simulink model "EmergencyBraking"  (R2023b)
settings: Solver=FixedStepAuto  StartTime=0.0  StopTime=inf  RelTol=1e-3
model workspace (MAT data in the model file):
  SL_ROS_VariableLengthArrays_MaxSizes.CommonInfo.ArrayTruncateAction = 'EmitWarning'
  SL_ROS_VariableLengthArrays_MaxSizes.MsgTypeMap = containers.Map
  SL_ROS_VariableLengthArrays_MaxSizes.MsgTypeMap.serialization.keys = {'sensor_msgs/PointCloud2'}
  SL_ROS_VariableLengthArrays_MaxSizes.MsgTypeMap.serialization.values{1}(1).PropertyName = 'data'
  SL_ROS_VariableLengthArrays_MaxSizes.MsgTypeMap.serialization.values{1}(1).DataType = 'uint8'
  SL_ROS_VariableLengthArrays_MaxSizes.MsgTypeMap.serialization.values{1}(1).MaxLength = 140000
  SL_ROS_VariableLengthArrays_MaxSizes.MsgTypeMap.serialization.values{1}(2).PropertyName = 'fields'
  SL_ROS_VariableLengthArrays_MaxSizes.MsgTypeMap.serialization.values{1}(2).DataType = 'sensor_msgs/PointField'
  SL_ROS_VariableLengthArrays_MaxSizes.MsgTypeMap.serialization.values{1}(2).MaxLength = 16
  SL_ROS_VariableLengthArrays_MaxSizes.MsgTypeMap.serialization.uniformity = 0
  SL_ROS_VariableLengthArrays_MaxSizes.MsgTypeMap.serialization.keyType = 'char'
  SL_ROS_VariableLengthArrays_MaxSizes.MsgTypeMap.serialization.valueType = 'any'
undefined symbols (not defined in the file): brake, throttle
libraries: ros2lib x5
settings Model: Creator=nikos  LastModifiedBy=nikos
settings OptimizationCC: EnhancedBackFolding=on  PassReuseOutputArgsAs=Individual arguments  ZeroExternalMemoryAtStartup=off  ZeroInternalMemoryAtStartup=off  MaxStackSize=64  OptimizeBlockOrder=speed  DifferentSizesBufferReuse=on  OptimizationCustomize=off  EfficientTunableParamExpr=on
settings DebuggingCC: ParameterTunabilityLossMsg=error
settings HardwareCC: ProdBitPerLong=64  ProdHWDeviceType=Intel->x86-64 (Linux 64)  UseEmbeddedCoderFeatures=off
settings SFSimCC: MATLABDynamicMemAlloc=off
settings RTWCC: Description=Embedded Coder  SystemTargetFile=ert.tlc  HardwareBoard=Robot Operating System 2 (ROS 2)  TLCOptions="-aInlineSetEventsForThisBaseRateFcn=TLC_FALSE -aSuppressMultiTaskScheduler=TLC_FALSE  -aRateBasedStepFcn=0"  TemplateMakefile=ert_default_tmf  Toolchain=Colcon Tools  TargetLang=C++
settings CodeAppCC: ForceParamTrailComments=on  IgnoreCustomStorageClasses=off  OperatorAnnotations=on  SimulinkDataObjDesc=on  SFDataObjDesc=on  InsertBlockDesc=on
settings ERTTargetCC: CodeInterfacePackaging=C++ class  SupportNonInlinedSFcns=on  RootIOFormat=Structure reference

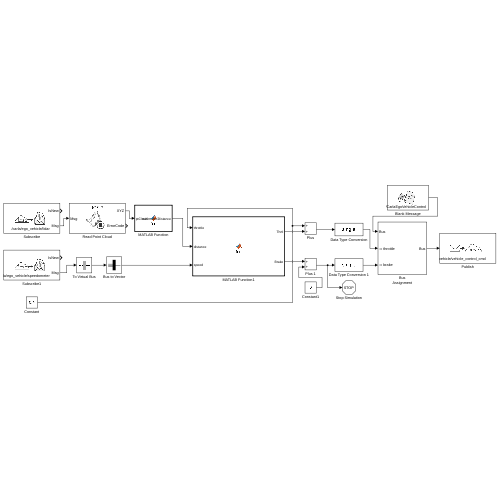
[thumbnail: Simulink's stored preview of the top-level diagram]
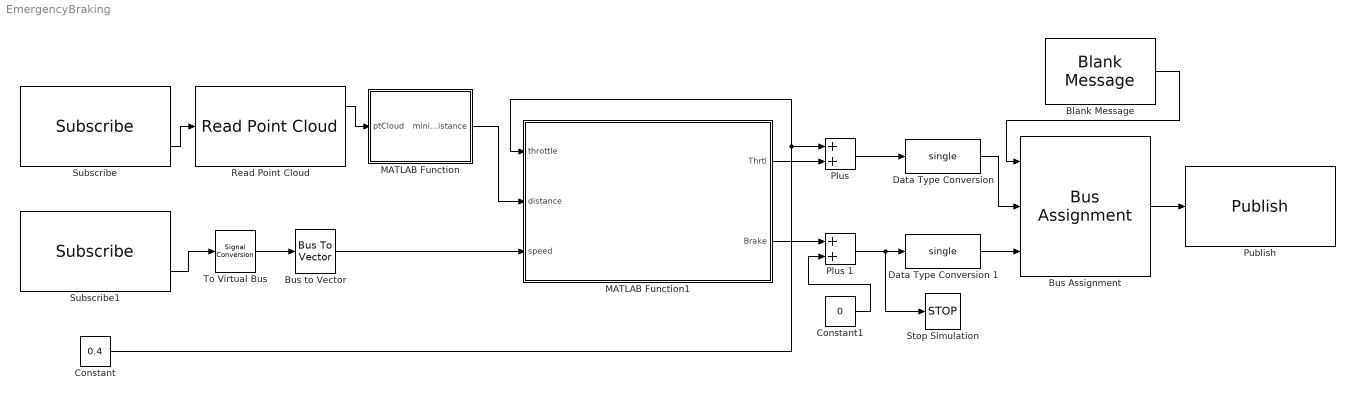
== system EmergencyBraking ==
  Blank Message : ros2lib/Blank Message  messageClass=Message  entityType=carla_msgs/CarlaEgoVehicleControl  messageType=carla_msgs/CarlaEgoVehicleControl  SampleTime=inf
  Bus Assignment : BusAssignment  AssignedSignals=throttle,brake
  Bus to Vector : BusToVector
  Constant : Constant  Value=0.4
  Constant1 : Constant  Value=0
  Data Type Conversion : DataTypeConversion  OutDataTypeStr=single  SaturateOnIntegerOverflow=off  RndMeth=Floor
  Data Type Conversion 1 : DataTypeConversion  OutDataTypeStr=single  SaturateOnIntegerOverflow=off  RndMeth=Floor
  MATLAB Function : MATLAB Function  TreatAsAtomicUnit=on
  MATLAB Function1 : MATLAB Function  TreatAsAtomicUnit=on
  Plus : Sum
  Plus 1 : Sum
  Publish : ros2lib/Publish  topicSource=Select from ROS network  topic=/carla/ego_vehicle/vehicle_control_cmd  messageType=carla_msgs/CarlaEgoVehicleControl  QOSHistory=Keep last  QOSDepth=1  QOSReliability=Reliable  QOSDurability=Volatile
  Read Point Cloud : ros2lib/Read Point Cloud  MaximumPointCloudSize=[480, 640]  PreserveStructure=off  ShowRGBOutput=off  ShowIntensityOutput=off  ShowErrorCodeOutput=on  VariableSizeOutputs=off
  Stop Simulation : Stop
  Subscribe : ros2lib/Subscribe  topicSource=Select from ROS network  topic=/carla/ego_vehicle/lidar  messageType=sensor_msgs/PointCloud2  sampleTime=-1  QOSHistory=Keep last  QOSDepth=1  QOSReliability=Reliable  QOSDurability=Volatile
  Subscribe1 : ros2lib/Subscribe  topicSource=Select from ROS network  topic=/carla/ego_vehicle/speedometer  messageType=std_msgs/Float32  sampleTime=-1  QOSHistory=Keep last  QOSDepth=1  QOSReliability=Reliable  QOSDurability=Volatile
  To Virtual Bus : SignalConversion  ConversionOutput=Virtual bus  OverrideOpt=off
  wires:
  Subscribe/2 -> Read Point Cloud/1
  Read Point Cloud/1 -> MATLAB Function/1(ptCloud)
  MATLAB Function/1(minimumXDistance) -> MATLAB Function1/2(distance)
  To Virtual Bus/1 -> Bus to Vector/1
  Subscribe1/2 -> To Virtual Bus/1
  Blank Message/1 -> Bus Assignment/1
  Bus Assignment/1 -> Publish/1
  Constant/1 -> MATLAB Function1/1(throttle), Plus/1
  Bus to Vector/1 -> MATLAB Function1/3(speed)
  MATLAB Function1/1(Thrtl) -> Plus/2
  MATLAB Function1/2(Brake) -> Plus 1/1
  Constant1/1 -> Plus 1/2
  Plus/1 -> Data Type Conversion/1
  Data Type Conversion/1 -> Bus Assignment/2
  Plus 1/1 -> Stop Simulation/1, Data Type Conversion 1/1
  Data Type Conversion 1/1 -> Bus Assignment/3

== matlab function EmergencyBraking/MATLAB Function1 ==
  data: throttle input; Thrtl output; distance input; speed input; Brake output
function [Thrtl, Brake] = fcn(throttle, distance, speed)

speed = speed * 3.6;

breakingDistance = (speed * speed) / (2 * 9.8 * 0.7 * 3.6 *3.6);

if distance > 0 && distance <= 2*breakingDistance
    Brake = 1;
    Thrtl = -throttle;
else
    Brake = 0 ;
    Thrtl = 0;

end

== matlab function EmergencyBraking/MATLAB Function ==
  data: minimumXDistance output; ptCloud input
function minimumXDistance  = fcn(ptCloud)

X = ptCloud(:,1);
Y = ptCloud(:,2);
Z = ptCloud(:,3);

ind = find(X>3 & Z>-2 & Y<2 & Y>-2);

Target_Data = [X(ind), Y(ind), Z(ind)];

xTarget = nonzeros(Target_Data(:,1));

minimumXDistance = 0.0;

if ~isempty(xTarget)
    minimumXDistance = double(min(xTarget)) - 2.4;

end
